simulink model "Passivity_based"  (R2019b)
settings: Solver=VariableStepAuto  StartTime=0.0  StopTime=10  FixedStep=.001  MaxStep=.1  RelTol=1e-3
settings Model: Creator=imi  LastModifiedBy=Ali Alaei
settings DataIOCC: ReturnWorkspaceOutputs=off
settings DebuggingCC: ArithmeticOperatorsInVariantConditions=warning
settings SFSimCC: SimUseLocalCustomCode=off  CustomCodeUndefinedFunction=UseInterfaceOnly
settings RTWCC: RTWUseLocalCustomCode=off
settings CodeAppCC: StateflowObjectComments=on

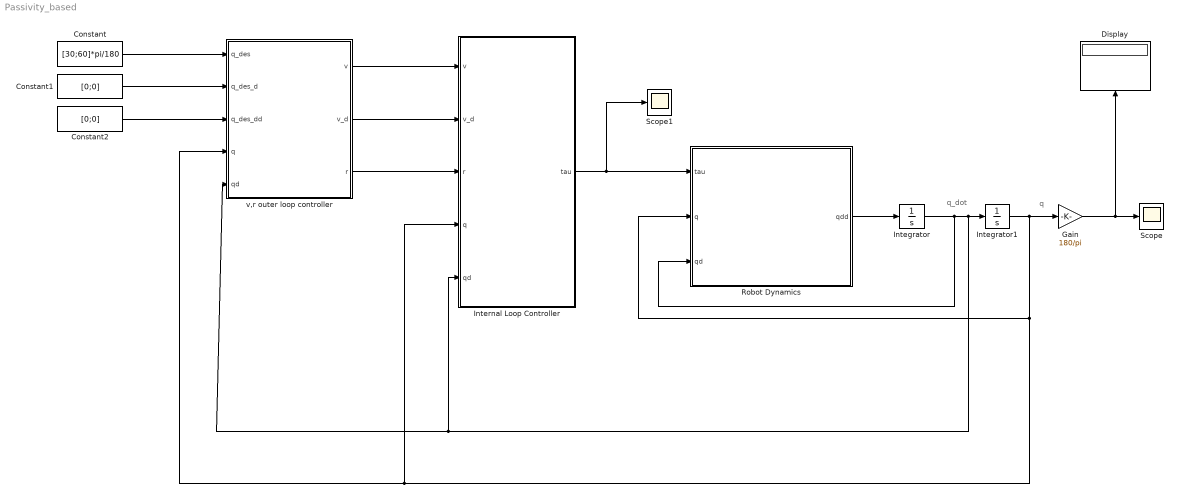
== system Passivity_based ==
  note: q
  note: q_dot
  Constant : Constant  Value=[30;60]*pi/180
  Constant1 : Constant  Value=[0;0]
  Constant2 : Constant  Value=[0;0]
  Display : Display
  Gain : Gain  Gain=180/pi
  Integrator : Integrator  InitialCondition=zeros(2,1)
  Integrator1 : Integrator  InitialCondition=[45;95]*pi/180*0
  Internal Loop Controller : MATLAB Function  TreatAsAtomicUnit=on
  Robot Dynamics : MATLAB Function  TreatAsAtomicUnit=on
  Scope : Scope
  Scope1 : Scope
  v,r outer loop controller : MATLAB Function  TreatAsAtomicUnit=on
  wires:
  Integrator/1 -> v,r outer loop controller/5(qd), Internal Loop Controller/5(qd), Integrator1/1, Robot Dynamics/3(qd)
  Robot Dynamics/1(qdd) -> Integrator/1
  Integrator1/1 -> v,r outer loop controller/4(q), Internal Loop Controller/4(q), Robot Dynamics/2(q), Gain/1
  Internal Loop Controller/1(tau) -> Scope1/1, Robot Dynamics/1(tau)
  Gain/1 -> Scope/1, Display/1
  Constant/1 -> v,r outer loop controller/1(q_des)
  Constant1/1 -> v,r outer loop controller/2(q_des_d)
  Constant2/1 -> v,r outer loop controller/3(q_des_dd)
  v,r outer loop controller/1(v) -> Internal Loop Controller/1(v)
  v,r outer loop controller/2(v_d) -> Internal Loop Controller/2(v_d)
  v,r outer loop controller/3(r) -> Internal Loop Controller/3(r)

== matlab function Passivity_based/Internal Loop Controller ==
  data: v input; v_d input; r input; q input; qd input; tau output
function tau = fcn(v,v_d,r,q,qd)

q1=q(1);
q2=q(2);

q1d=qd(1);
q2d=qd(2);




m1=2;
m2=1.4;

I1=.5;
I2=.1;

l1=.8;
l2=.8;

lc1=.4;
lc2=.4;


g=9.81;



d11=m1*lc1^2+I1+I2+m2*(l1^2+lc2^2+2*l1*lc2*cos(q2));
d12=m2*lc2^2+I2+m2*l2*lc2*cos(q2);
d21=m2*lc2^2+I2+m2*l2*lc2*cos(q2);
d22=m2*lc2^2+I2;

c11=-m2*l1*lc2*sin(q2)*q2d;
c12=-m2*l1*lc2*sin(q2)*(q1d+q2d);
c21=m2*l1*lc2*sin(q2)*q1d;
c22=0;

g11=m1*lc1*g*cos(q1)+m2*g*(lc2*cos(q1+q2)+l1*cos(q1));
g21=m2*lc2*g*cos(q1+q2);

M=[d11,d12;d21,d22];
C=[c11 c12;c21 c22];
G=[g11;g21];
K=21*eye(2);

tau=M*v_d+C*v+G-K*r;

== matlab function Passivity_based/Robot Dynamics ==
  data: tau input; q input; qdd output; qd input
function qdd = fcn(tau,q,qd)

q1=q(1);
q2=q(2);

q1d=qd(1);
q2d=qd(2);




m1=2;
m2=1.4;

I1=.5;
I2=.1;

l1=.8;
l2=.8;

lc1=.4;
lc2=.4;


g=9.81;



d11=m1*lc1^2+I1+I2+m2*(l1^2+lc2^2+2*l1*lc2*cos(q2));
d12=m2*lc2^2+I2+m2*l2*lc2*cos(q2);
d21=m2*lc2^2+I2+m2*l2*lc2*cos(q2);
d22=m2*lc2^2+I2;

c11=-m2*l1*lc2*sin(q2)*q2d;
c12=-m2*l1*lc2*sin(q2)*(q1d+q2d);
c21=m2*l1*lc2*sin(q2)*q1d;
c22=0;

g11=m1*lc1*g*cos(q1)+m2*g*(lc2*cos(q1+q2)+l1*cos(q1));
g21=m2*lc2*g*cos(q1+q2);

M=[d11,d12;d21,d22];
C=[c11 c12;c21 c22];
G=[g11;g21];
qdd=pinv(M)*(tau-C*qd-G);

== matlab function Passivity_based/v,r outer loop controller ==
  data: q_des input; q_des_d input; q_des_dd input; q input; qd input; v output; v_d output; r output
function [v,v_d,r]= fcn(q_des,q_des_d,q_des_dd,q,qd)


q_tilde=q-q_des;
q_tilde_d=qd-q_des_d;

gamma=15;


v=q_des_d-gamma*q_tilde;
v_d=q_des_dd-gamma*q_tilde_d;
r=qd-v;
